simulink subsystem "KScale"  (R2021b)
settings: Solver=VariableStepAuto  StartTime=0.0  StopTime=10.0  RelTol=1e-3
undefined symbols (not defined in the file): solubilityScale
settings Model: Creator=Jiaqi  LastModifiedBy=Jiaqi

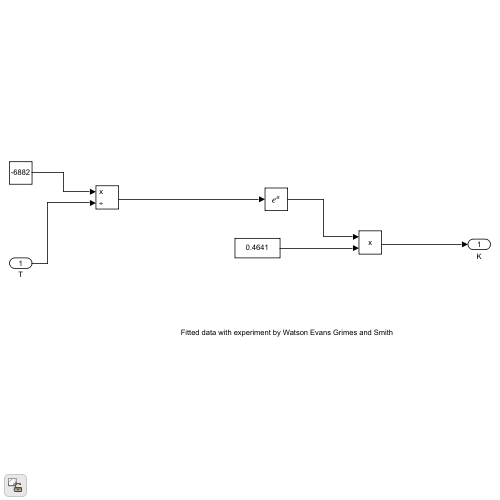
[thumbnail: Simulink's stored preview of the top-level diagram]
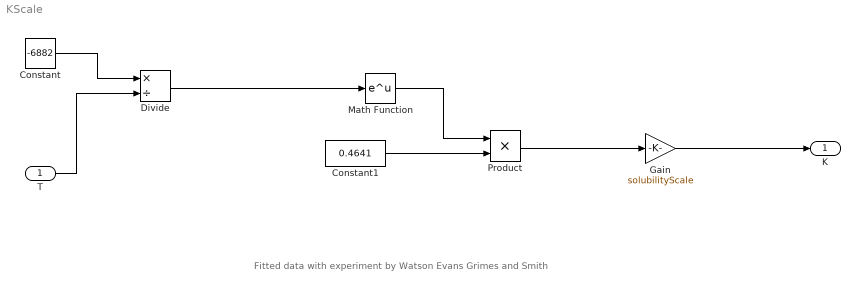
== system KScale ==
  note: Fitted data with experiment by Watson Evans Grimes and Smith
  T : Inport
  Constant : Constant  Value=-6882
  Constant1 : Constant  Value=0.4641
  Divide : Product  Inputs=*/
  Gain : Gain  Gain=solubilityScale
  Math Function : Math  SaturateOnIntegerOverflow=on
  Product : Product
  K : Outport
  wires:
  Constant/1 -> Divide/1
  T/1 -> Divide/2
  Divide/1 -> Math Function/1
  Math Function/1 -> Product/1
  Constant1/1 -> Product/2
  Product/1 -> Gain/1
  Gain/1 -> K/1
